simulink model "rotpendirect"  (R2024b)
settings: Solver=VariableStepAuto  StartTime=0.0  StopTime=10.0  RelTol=1e-3
values from neighbouring files (symbols this model uses):
  cA = [0 0 1 0 ... (first row only)    [inverted_rotary_pendulum.m]    (also in rotaryPendulum.m)
  cB = Kg * kt * cB / Rm    [inverted_rotary_pendulum.m]    (also in rotaryPendulum.m)
  cI = eye(size(cA))    [inverted_rotary_pendulum.m]
  cO = 0*cB    [inverted_rotary_pendulum.m]
  Ts = 0.05    [inverted_rotary_pendulum.m]    (also in rotaryPendulum.m = 0.01)
  x0 = [0; 0.174; 0; 0.767]    [inverted_rotary_pendulum.m]    (also in rotaryPendulum.m)
undefined symbols (not defined in the file or in its folder): K
settings Model: Creator=yu  LastModifiedBy=yu

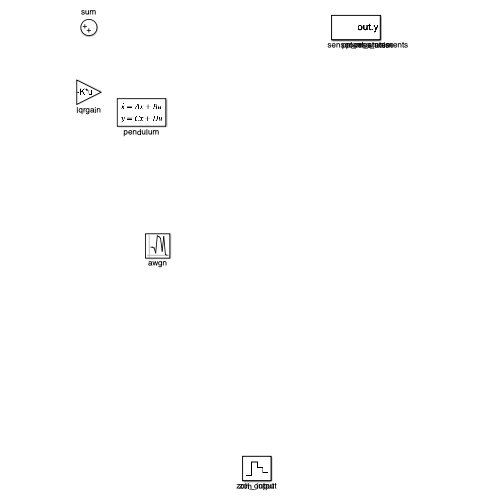
[thumbnail: Simulink's stored preview of the top-level diagram]
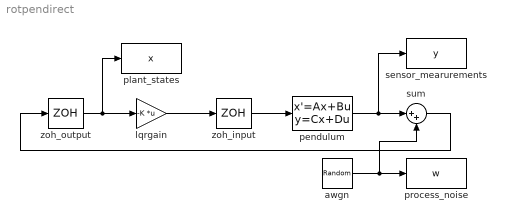
== system rotpendirect ==
  awgn : RandomNumber  Variance=2.5e-9  SampleTime=Ts
  lqrgain : Gain  Gain=-K  Multiplication=Matrix(K*u)
  pendulum : StateSpace  A=cA  B=cB  C=cI  D=cO  InitialCondition=x0
  plant_states : ToWorkspace  VariableName=x  SaveFormat=Timeseries  SampleTime=-1
  process_noise : ToWorkspace  VariableName=w  SaveFormat=Timeseries  SampleTime=-1
  sensor_mearurements : ToWorkspace  VariableName=y  SaveFormat=Timeseries  SampleTime=-1
  sum : Sum  Inputs=|++
  zoh_input : ZeroOrderHold  SampleTime=-1
  zoh_output : ZeroOrderHold  SampleTime=-1
  wires:
  sum/1 -> zoh_output/1
  lqrgain/1 -> zoh_input/1
  awgn/1 -> process_noise/1, sum/2
  pendulum/1 -> sensor_mearurements/1, sum/1
  zoh_input/1 -> pendulum/1
  zoh_output/1 -> lqrgain/1, plant_states/1
